simulink model "RealtimeModel"  (Simulink 7.0)
settings: Solver=FixedStepDiscrete  SolverMode=MultiTasking  StartTime=0.0  StopTime=RunningTime  FixedStep=sample  RelTol=1e-3
values from neighbouring files (symbols this model uses):
  Integrator = InitializeIntegrator(Integrator, Structure)    [RealtimeModel_Setup.m]
  Interpolations = SampleRate/sample    [RealtimeModel_Setup.m]
  sample = 1/1024    (= 0.0009765625)    [RealtimeModel_Setup.m]
  SampleRate = Integrator.Timestep    [RealtimeModel_Setup.m]
undefined symbols (not defined in the file or in its folder): Elements
(part 1 of 3)
CloseFcn:
  | rtwprivate ssgencode ModelCloseRequest hybriddaq1dof
settings Model: MinMaxOverflowLogging=ForceOff  Creator=NEESsim1  LastModifiedBy=Tommy  BufferReuse=off
settings OptimizationCC: BlockReduction=off  OptimizeBlockIOStorage=off  BufferReuse=off  ExpressionFolding=off  LocalBlockOutputs=off
settings DebuggingCC: SignalResolutionControl=TryResolveAllWithWarning  MultiTaskDSMMsg=warning  StrictBusMsg=ErrorLevel1
settings RTWCC: SystemTargetFile=xpctarget.tlc  TemplateMakefile=xpc_default_tmf  Description=xPC Target  ProcessScript=xpctarget_make_rtw_hook
settings xpcTargetCC: TargetFcnLib=ansi_tfl_tmw.mat  GenFloatMathFcnCalls=ANSI_C  CompOptLevelCompliant=off  PortableWordSizes=off
settings CustomProperty: DataType=string  Value=Real-Time

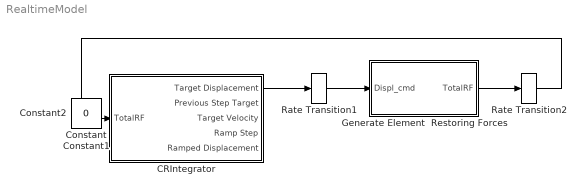
== system RealtimeModel ==
  CRIntegrator : Subsystem
  Generate Element  Restoring Forces : Subsystem  TreatAsAtomicUnit=on  SystemSampleTime=SampleRate
  Rate Transition1 : RateTransition  Deterministic=off
  Rate Transition2 : RateTransition  Deterministic=off
  Constant : Constant  IOType=siggen  Value=0  OutDataType=sfix(16)  OutScaling=2^0
  Constant1 : Constant  IOType=siggen  Value=0  OutDataType=sfix(16)  OutScaling=2^0
  Constant2 : Constant  IOType=siggen  Value=0  OutDataType=sfix(16)  OutScaling=2^0
  wires:
  Rate Transition1/1 -> Generate Element  Restoring Forces/1(Displ_cmd)
  Generate Element  Restoring Forces/1(TotalRF) -> Rate Transition2/1
  CRIntegrator/1(Target Displacement) -> Rate Transition1/1
  Rate Transition2/1 -> CRIntegrator/1(TotalRF)

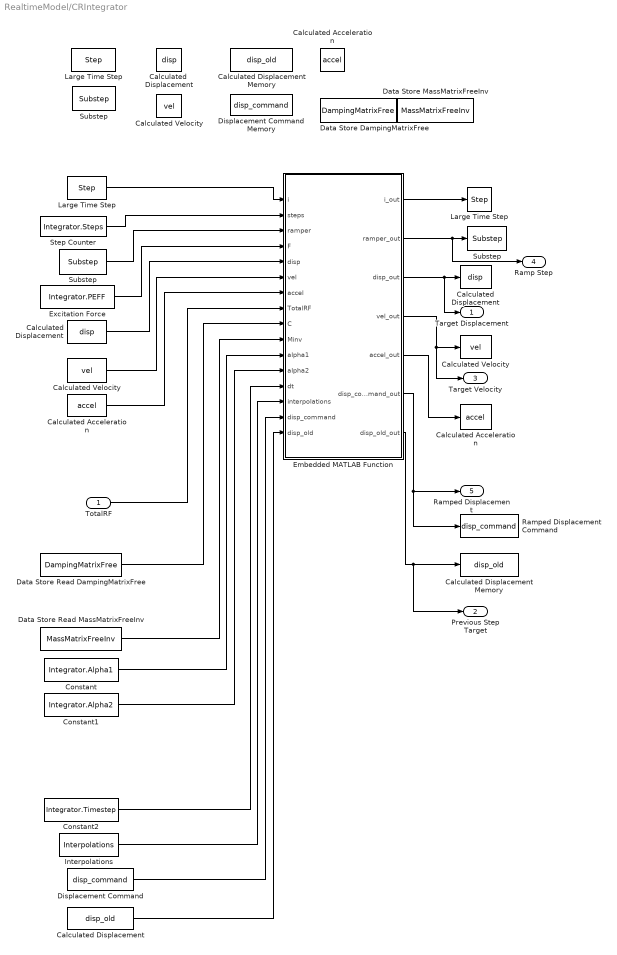
== system RealtimeModel/CRIntegrator ==
  TotalRF : Inport  OutDataType=sfix(16)  OutScaling=2^0
  " Calculated Acceleration" : DataStoreWrite  DataStoreName=accel  SampleTime=sample
  " Calculated Displacement" : DataStoreWrite  DataStoreName=disp  SampleTime=sample
  " Calculated Displacement Memory" : DataStoreWrite  DataStoreName=disp_old  SampleTime=sample
  " Calculated Velocity" : DataStoreWrite  DataStoreName=vel  SampleTime=sample
  " Large Time Step" : DataStoreWrite  DataStoreName=Step  SampleTime=sample
  " Substep" : DataStoreWrite  DataStoreName=Substep  SampleTime=sample
  Calculated Acceleration : DataStoreMemory  DataStoreName=accel  InitialValue=Integrator.Acceleration  OutDataType=sfix(16)  OutScaling=2^0
  Calculated Velocity : DataStoreMemory  DataStoreName=vel  InitialValue=Integrator.Velocity  OutDataType=sfix(16)  OutScaling=2^0
  Calculated  Displacement : DataStoreMemory  DataStoreName=disp  InitialValue=Integrator.Displacement  OutDataType=sfix(16)  OutScaling=2^0
  "Calculated Acceleration " : DataStoreRead  DataStoreName=accel  SampleTime=sample
  Calculated Displacement : DataStoreRead  DataStoreName=disp_old  SampleTime=sample
  Calculated Displacement Memory : DataStoreMemory  DataStoreName=disp_old  InitialValue=Integrator.Displacement  OutDataType=sfix(16)  OutScaling=2^0
  "Calculated Displacement " : DataStoreRead  DataStoreName=disp  SampleTime=sample
  "Calculated Velocity " : DataStoreRead  DataStoreName=vel  SampleTime=sample
  Constant : Constant  Value=Integrator.Alpha1  OutDataType=sfix(16)  OutScaling=2^0
  Constant1 : Constant  Value=Integrator.Alpha2  OutDataType=sfix(16)  OutScaling=2^0
  Constant2 : Constant  Value=Integrator.Timestep  OutDataType=sfix(16)  OutScaling=2^0
  Data Store DampingMatrixFree : DataStoreMemory  DataStoreName=DampingMatrixFree  InitialValue=Structure.DampingMatrixFree  OutDataType=sfix(16)  OutScaling=2^0
  Data Store MassMatrixFreeInv : DataStoreMemory  DataStoreName=MassMatrixFreeInv  InitialValue=Structure.MassMatrixFreeInv  OutDataType=sfix(16)  OutScaling=2^0
  Data Store Read DampingMatrixFree : DataStoreRead  DataStoreName=DampingMatrixFree  SampleTime=sample
  Data Store Read MassMatrixFreeInv : DataStoreRead  DataStoreName=MassMatrixFreeInv  SampleTime=sample
  Displacement Command Memory : DataStoreMemory  DataStoreName=disp_command  InitialValue=Integrator.Displacement  OutDataType=sfix(16)  OutScaling=2^0
  "Displacement Command " : DataStoreRead  DataStoreName=disp_command  SampleTime=sample
  Embedded MATLAB Function : Stateflow chart
  Excitation Force : Constant  Value=Integrator.PEFF  OutDataType=sfix(16)  OutScaling=2^0
  Interpolations : Constant  Value=Interpolations  OutDataType=sfix(16)  OutScaling=2^0  SampleTime=sample
  Large Time Step : DataStoreMemory  DataStoreName=Step  OutDataType=sfix(16)  OutScaling=2^0
  "Large Time Step " : DataStoreRead  DataStoreName=Step  SampleTime=sample
  Ramped Displacement Command : DataStoreWrite  DataStoreName=disp_command  SampleTime=sample
  Step Counter : Constant  Value=Integrator.Steps  OutDataType=sfix(16)  OutScaling=2^0  SampleTime=sample
  Substep : DataStoreMemory  DataStoreName=Substep  InitialValue=1  OutDataType=sfix(16)  OutScaling=2^0
  "Substep " : DataStoreRead  DataStoreName=Substep  SampleTime=sample
  Target Displacement : Outport  OutDataType=sfix(16)  OutScaling=2^0
  Previous Step Target : Outport  Port=2  OutDataType=sfix(16)  OutScaling=2^0
  Target Velocity : Outport  Port=3  OutDataType=sfix(16)  OutScaling=2^0
  Ramp Step : Outport  Port=4  OutDataType=sfix(16)  OutScaling=2^0
  Ramped Displacement : Outport  Port=5  OutDataType=sfix(16)  OutScaling=2^0
  wires:
  Excitation Force/1 -> Embedded MATLAB Function/4(F)
  Calculated Displacement/1 -> Embedded MATLAB Function/16(disp_old)
  "Displacement Command "/1 -> Embedded MATLAB Function/15(disp_command)
  "Calculated Acceleration "/1 -> Embedded MATLAB Function/7(accel)
  "Calculated Velocity "/1 -> Embedded MATLAB Function/6(vel)
  "Calculated Displacement "/1 -> Embedded MATLAB Function/5(disp)
  "Substep "/1 -> Embedded MATLAB Function/3(ramper)
  Embedded MATLAB Function/7(disp_old_out) -> Previous Step Target/1, " Calculated Displacement Memory"/1
  Embedded MATLAB Function/5(accel_out) -> " Calculated Acceleration"/1
  Embedded MATLAB Function/3(disp_out) -> " Calculated Displacement"/1, Target Displacement/1
  Embedded MATLAB Function/2(ramper_out) -> Ramp Step/1, " Substep"/1
  Embedded MATLAB Function/1(i_out) -> " Large Time Step"/1
  Constant1/1 -> Embedded MATLAB Function/12(alpha2)
  Constant/1 -> Embedded MATLAB Function/11(alpha1)
  Step Counter/1 -> Embedded MATLAB Function/2(steps)
  Constant2/1 -> Embedded MATLAB Function/13(dt)
  TotalRF/1 -> Embedded MATLAB Function/8(TotalRF)
  Embedded MATLAB Function/6(disp_command_out) -> Ramped Displacement Command/1, Ramped Displacement/1
  Embedded MATLAB Function/4(vel_out) -> " Calculated Velocity"/1, Target Velocity/1
  Interpolations/1 -> Embedded MATLAB Function/14(interpolations)
  Data Store Read MassMatrixFreeInv/1 -> Embedded MATLAB Function/10(Minv)
  Data Store Read DampingMatrixFree/1 -> Embedded MATLAB Function/9(C)
  "Large Time Step "/1 -> Embedded MATLAB Function/1(i)

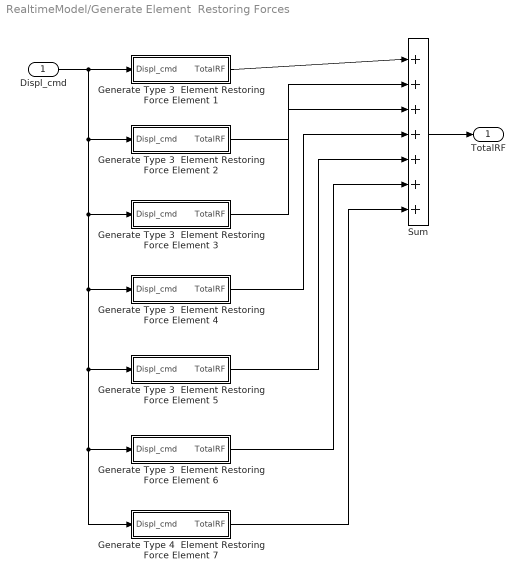
== system RealtimeModel/Generate Element  Restoring Forces ==
  Displ_cmd : Inport  OutDataType=sfix(16)  OutScaling=2^0
  Generate Type 3  Element Restoring Force Element 1 : Subsystem  TreatAsAtomicUnit=on  SystemSampleTime=SampleRate  mask(Generate Type 3 Element Restoring Force){id=1}
      mask prompts: id "Element ID"
      mask help:
      | Generates the Restoring Force vector for a Type 3 Element
      |
      | Enter the ID for this element corresponding with the input configuration file
  Generate Type 3  Element Restoring Force Element 2 : Subsystem  TreatAsAtomicUnit=on  SystemSampleTime=SampleRate  mask(Generate Type 3 Element Restoring Force){id=2}
      mask prompts: id "Element ID"
      mask help:
      | Generates the Restoring Force vector for a Type 3 Element
      |
      | Enter the ID for this element corresponding with the input configuration file
  Generate Type 3  Element Restoring Force Element 3 : Subsystem  TreatAsAtomicUnit=on  SystemSampleTime=SampleRate  mask(Generate Type 3 Element Restoring Force){id=3}
      mask prompts: id "Element ID"
      mask help:
      | Generates the Restoring Force vector for a Type 3 Element
      |
      | Enter the ID for this element corresponding with the input configuration file
  Generate Type 3  Element Restoring Force Element 4 : Subsystem  TreatAsAtomicUnit=on  SystemSampleTime=SampleRate  mask(Generate Type 3 Element Restoring Force){id=4}
      mask prompts: id "Element ID"
      mask help:
      | Generates the Restoring Force vector for a Type 3 Element
      |
      | Enter the ID for this element corresponding with the input configuration file
  Generate Type 3  Element Restoring Force Element 5 : Subsystem  TreatAsAtomicUnit=on  SystemSampleTime=SampleRate  mask(Generate Type 3 Element Restoring Force){id=5}
      mask prompts: id "Element ID"
      mask help:
      | Generates the Restoring Force vector for a Type 3 Element
      |
      | Enter the ID for this element corresponding with the input configuration file
  Generate Type 3  Element Restoring Force Element 6 : Subsystem  TreatAsAtomicUnit=on  SystemSampleTime=SampleRate  mask(Generate Type 3 Element Restoring Force){id=6}
      mask prompts: id "Element ID"
      mask help:
      | Generates the Restoring Force vector for a Type 3 Element
      |
      | Enter the ID for this element corresponding with the input configuration file
  Generate Type 4  Element Restoring Force Element 7 : Subsystem  TreatAsAtomicUnit=on  SystemSampleTime=SampleRate  mask(Generate Type 4 Element Restoring Force){id=7}
      mask prompts: id "Element ID"
      mask help:
      | Generates the Restoring Force vector for a Type 4 Element
      |
      | Enter the ID for this element corresponding with the input configuration file
  Sum : Sum  Inputs=|+++++++  OutDataType=sfix(16)  OutScaling=2^0
  TotalRF : Outport  OutDataType=sfix(16)  OutScaling=2^0
  wires:
  Displ_cmd/1 -> Generate Type 3  Element Restoring Force Element 1/1(Displ_cmd), Generate Type 3  Element Restoring Force Element 2/1(Displ_cmd), Generate Type 3  Element Restoring Force Element 3/1(Displ_cmd), Generate Type 3  Element Restoring Force Element 4/1(Displ_cmd), Generate Type 3  Element Restoring Force Element 5/1(Displ_cmd), Generate Type 3  Element Restoring Force Element 6/1(Displ_cmd), Generate Type 4  Element Restoring Force Element 7/1(Displ_cmd)
  Sum/1 -> TotalRF/1
  Generate Type 3  Element Restoring Force Element 1/1(TotalRF) -> Sum/1
  Generate Type 3  Element Restoring Force Element 2/1(TotalRF) -> Sum/2
  Generate Type 3  Element Restoring Force Element 3/1(TotalRF) -> Sum/3
  Generate Type 3  Element Restoring Force Element 4/1(TotalRF) -> Sum/4
  Generate Type 3  Element Restoring Force Element 5/1(TotalRF) -> Sum/5
  Generate Type 3  Element Restoring Force Element 6/1(TotalRF) -> Sum/6
  Generate Type 4  Element Restoring Force Element 7/1(TotalRF) -> Sum/7

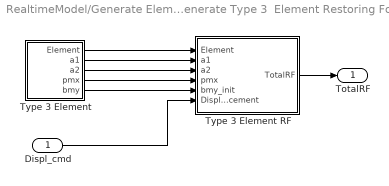
== system RealtimeModel/Generate Element  Restoring Forces/Generate Type 3  Element Restoring Force Element 1 ==
  Displ_cmd : Inport  OutDataType=sfix(16)  OutScaling=2^0
  "Type 3 Element " : Subsystem  mask(Element Type 3){id=id}
      mask prompts: id "Element ID:"
      mask help: Enter the ID for this element corresponding with the input configuration file
  Type 3 Element RF : Stateflow chart  TreatAsAtomicUnit=on  SystemSampleTime=SampleRate
  TotalRF : Outport  OutDataType=sfix(16)  OutScaling=2^0
  wires:
  Displ_cmd/1 -> Type 3 Element RF/6(Displacement)
  "Type 3 Element "/1(Element) -> Type 3 Element RF/1(Element)
  Type 3 Element RF/1(TotalRF) -> TotalRF/1
  "Type 3 Element "/2(a1) -> Type 3 Element RF/2(a1)
  "Type 3 Element "/3(a2) -> Type 3 Element RF/3(a2)
  "Type 3 Element "/4(pmx) -> Type 3 Element RF/4(pmx)
  "Type 3 Element "/5(bmy) -> Type 3 Element RF/5(bmy_init)

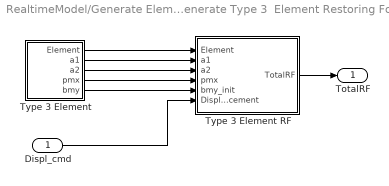
== system RealtimeModel/Generate Element  Restoring Forces/Generate Type 3  Element Restoring Force Element 2 ==
  Displ_cmd : Inport  OutDataType=sfix(16)  OutScaling=2^0
  "Type 3 Element " : Subsystem  mask(Element Type 3){id=id}
      mask prompts: id "Element ID:"
      mask help: Enter the ID for this element corresponding with the input configuration file
  Type 3 Element RF : Stateflow chart  TreatAsAtomicUnit=on  SystemSampleTime=SampleRate
  TotalRF : Outport  OutDataType=sfix(16)  OutScaling=2^0
  wires:
  "Type 3 Element "/5(bmy) -> Type 3 Element RF/5(bmy_init)
  "Type 3 Element "/4(pmx) -> Type 3 Element RF/4(pmx)
  "Type 3 Element "/3(a2) -> Type 3 Element RF/3(a2)
  "Type 3 Element "/2(a1) -> Type 3 Element RF/2(a1)
  Type 3 Element RF/1(TotalRF) -> TotalRF/1
  "Type 3 Element "/1(Element) -> Type 3 Element RF/1(Element)
  Displ_cmd/1 -> Type 3 Element RF/6(Displacement)

== system RealtimeModel/Generate Element  Restoring Forces/Generate Type 3  Element Restoring Force Element 3 ==
  Displ_cmd : Inport  OutDataType=sfix(16)  OutScaling=2^0
  "Type 3 Element " : Subsystem  mask(Element Type 3){id=id}
      mask prompts: id "Element ID:"
      mask help: Enter the ID for this element corresponding with the input configuration file
  Type 3 Element RF : Stateflow chart  TreatAsAtomicUnit=on  SystemSampleTime=SampleRate
  TotalRF : Outport  OutDataType=sfix(16)  OutScaling=2^0
  wires:
  "Type 3 Element "/5(bmy) -> Type 3 Element RF/5(bmy_init)
  "Type 3 Element "/4(pmx) -> Type 3 Element RF/4(pmx)
  "Type 3 Element "/3(a2) -> Type 3 Element RF/3(a2)
  "Type 3 Element "/2(a1) -> Type 3 Element RF/2(a1)
  Type 3 Element RF/1(TotalRF) -> TotalRF/1
  "Type 3 Element "/1(Element) -> Type 3 Element RF/1(Element)
  Displ_cmd/1 -> Type 3 Element RF/6(Displacement)

== system RealtimeModel/Generate Element  Restoring Forces/Generate Type 3  Element Restoring Force Element 4 ==
  Displ_cmd : Inport  OutDataType=sfix(16)  OutScaling=2^0
  "Type 3 Element " : Subsystem  mask(Element Type 3){id=id}
      mask prompts: id "Element ID:"
      mask help: Enter the ID for this element corresponding with the input configuration file
  Type 3 Element RF : Stateflow chart  TreatAsAtomicUnit=on  SystemSampleTime=SampleRate
  TotalRF : Outport  OutDataType=sfix(16)  OutScaling=2^0
  wires:
  Displ_cmd/1 -> Type 3 Element RF/6(Displacement)
  "Type 3 Element "/1(Element) -> Type 3 Element RF/1(Element)
  Type 3 Element RF/1(TotalRF) -> TotalRF/1
  "Type 3 Element "/2(a1) -> Type 3 Element RF/2(a1)
  "Type 3 Element "/3(a2) -> Type 3 Element RF/3(a2)
  "Type 3 Element "/4(pmx) -> Type 3 Element RF/4(pmx)
  "Type 3 Element "/5(bmy) -> Type 3 Element RF/5(bmy_init)

== system RealtimeModel/Generate Element  Restoring Forces/Generate Type 3  Element Restoring Force Element 5 ==
  Displ_cmd : Inport  OutDataType=sfix(16)  OutScaling=2^0
  "Type 3 Element " : Subsystem  mask(Element Type 3){id=id}
      mask prompts: id "Element ID:"
      mask help: Enter the ID for this element corresponding with the input configuration file
  Type 3 Element RF : Stateflow chart  TreatAsAtomicUnit=on  SystemSampleTime=SampleRate
  TotalRF : Outport  OutDataType=sfix(16)  OutScaling=2^0
  wires:
  "Type 3 Element "/5(bmy) -> Type 3 Element RF/5(bmy_init)
  "Type 3 Element "/4(pmx) -> Type 3 Element RF/4(pmx)
  "Type 3 Element "/3(a2) -> Type 3 Element RF/3(a2)
  "Type 3 Element "/2(a1) -> Type 3 Element RF/2(a1)
  Type 3 Element RF/1(TotalRF) -> TotalRF/1
  "Type 3 Element "/1(Element) -> Type 3 Element RF/1(Element)
  Displ_cmd/1 -> Type 3 Element RF/6(Displacement)

== system RealtimeModel/Generate Element  Restoring Forces/Generate Type 3  Element Restoring Force Element 6 ==
  Displ_cmd : Inport  OutDataType=sfix(16)  OutScaling=2^0
  "Type 3 Element " : Subsystem  mask(Element Type 3){id=id}
      mask prompts: id "Element ID:"
      mask help: Enter the ID for this element corresponding with the input configuration file
  Type 3 Element RF : Stateflow chart  TreatAsAtomicUnit=on  SystemSampleTime=SampleRate
  TotalRF : Outport  OutDataType=sfix(16)  OutScaling=2^0
  wires:
  Displ_cmd/1 -> Type 3 Element RF/6(Displacement)
  "Type 3 Element "/1(Element) -> Type 3 Element RF/1(Element)
  Type 3 Element RF/1(TotalRF) -> TotalRF/1
  "Type 3 Element "/2(a1) -> Type 3 Element RF/2(a1)
  "Type 3 Element "/3(a2) -> Type 3 Element RF/3(a2)
  "Type 3 Element "/4(pmx) -> Type 3 Element RF/4(pmx)
  "Type 3 Element "/5(bmy) -> Type 3 Element RF/5(bmy_init)

== system RealtimeModel/Generate Element  Restoring Forces/Generate Type 4  Element Restoring Force Element 7 ==
  Displ_cmd : Inport  OutDataType=sfix(16)  OutScaling=2^0
  "Type 4 Element " : Subsystem  mask(Element Type 4){id=id}
      mask prompts: id "Element ID:"
      mask help: Enter the ID for this element corresponding with the input configuration file
  Type 4 Element RF : Stateflow chart  TreatAsAtomicUnit=on  SystemSampleTime=SampleRate
  TotalRF : Outport  OutDataType=sfix(16)  OutScaling=2^0
  wires:
  "Type 4 Element "/1(Element) -> Type 4 Element RF/1(Element)
  Type 4 Element RF/1(TotalRF) -> TotalRF/1
  Displ_cmd/1 -> Type 4 Element RF/2(Displacement)

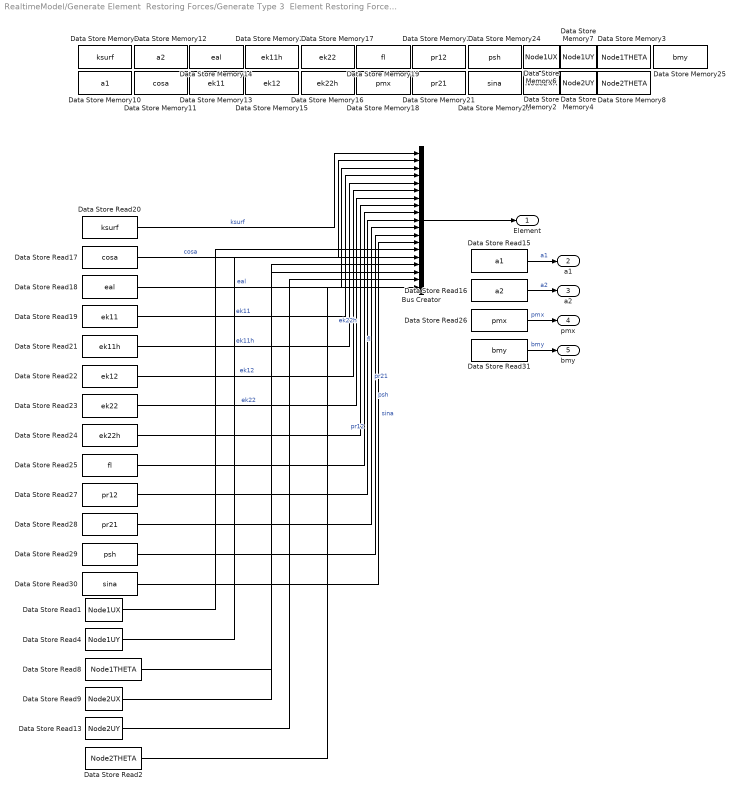
== system RealtimeModel/Generate Element  Restoring Forces/Generate Type 3  Element Restoring Force Element 1/Type 3 Element  ==
  Bus Creator : BusCreator  Inputs=19
  Data Store Memory10 : DataStoreMemory  DataStoreName=a1  InitialValue=Elements{id}.a1  OutDataType=sfix(16)  OutScaling=2^0
  Data Store Memory11 : DataStoreMemory  DataStoreName=cosa  InitialValue=Elements{id}.cosa  OutDataType=sfix(16)  OutScaling=2^0
  Data Store Memory12 : DataStoreMemory  DataStoreName=a2  InitialValue=Elements{id}.a2  OutDataType=sfix(16)  OutScaling=2^0
  Data Store Memory13 : DataStoreMemory  DataStoreName=ek11  InitialValue=Elements{id}.ek11  OutDataType=sfix(16)  OutScaling=2^0
  Data Store Memory14 : DataStoreMemory  DataStoreName=eal  InitialValue=Elements{id}.eal  OutDataType=sfix(16)  OutScaling=2^0
  Data Store Memory15 : DataStoreMemory  DataStoreName=ek12  InitialValue=Elements{id}.ek12  OutDataType=sfix(16)  OutScaling=2^0
  Data Store Memory16 : DataStoreMemory  DataStoreName=ek22h  InitialValue=Elements{id}.ek22h  OutDataType=sfix(16)  OutScaling=2^0
  Data Store Memory17 : DataStoreMemory  DataStoreName=ek22  InitialValue=Elements{id}.ek22  OutDataType=sfix(16)  OutScaling=2^0
  Data Store Memory18 : DataStoreMemory  DataStoreName=pmx  InitialValue=Elements{id}.pmx  OutDataType=sfix(16)  OutScaling=2^0
  Data Store Memory19 : DataStoreMemory  DataStoreName=fl  InitialValue=Elements{id}.fl  OutDataType=sfix(16)  OutScaling=2^0
  Data Store Memory2 : DataStoreMemory  DataStoreName=Node2UX  InitialValue=Elements{id}.Nodes(2).UX  OutDataType=sfix(16)  OutScaling=2^0
  Data Store Memory20 : DataStoreMemory  DataStoreName=ek11h  InitialValue=Elements{id}.ek11h  OutDataType=sfix(16)  OutScaling=2^0
  Data Store Memory21 : DataStoreMemory  DataStoreName=pr21  InitialValue=Elements{id}.pr21  OutDataType=sfix(16)  OutScaling=2^0
  Data Store Memory22 : DataStoreMemory  DataStoreName=pr12  InitialValue=Elements{id}.pr12  OutDataType=sfix(16)  OutScaling=2^0
  Data Store Memory23 : DataStoreMemory  DataStoreName=sina  InitialValue=Elements{id}.sina  OutDataType=sfix(16)  OutScaling=2^0
  Data Store Memory24 : DataStoreMemory  DataStoreName=psh  InitialValue=Elements{id}.psh  OutDataType=sfix(16)  OutScaling=2^0
  Data Store Memory25 : DataStoreMemory  DataStoreName=bmy  InitialValue=Elements{id}.bmy  OutDataType=sfix(16)  OutScaling=2^0
  Data Store Memory3 : DataStoreMemory  DataStoreName=Node1THETA  InitialValue=Elements{id}.Nodes(1).THETA  OutDataType=sfix(16)  OutScaling=2^0
  Data Store Memory4 : DataStoreMemory  DataStoreName=Node2UY  InitialValue=Elements{id}.Nodes(2).UY  OutDataType=sfix(16)  OutScaling=2^0
  Data Store Memory6 : DataStoreMemory  DataStoreName=Node1UX  InitialValue=Elements{id}.Nodes(1).UX  OutDataType=sfix(16)  OutScaling=2^0
  Data Store Memory7 : DataStoreMemory  DataStoreName=Node1UY  InitialValue=Elements{id}.Nodes(1).UY  OutDataType=sfix(16)  OutScaling=2^0
  Data Store Memory8 : DataStoreMemory  DataStoreName=Node2THETA  InitialValue=Elements{id}.Nodes(2).THETA  OutDataType=sfix(16)  OutScaling=2^0
  Data Store Memory9 : DataStoreMemory  DataStoreName=ksurf  InitialValue=Elements{id}.ksurf  OutDataType=sfix(16)  OutScaling=2^0
  Data Store Read1 : DataStoreRead  DataStoreName=Node1UX  SampleTime=-1
  Data Store Read13 : DataStoreRead  DataStoreName=Node2UY  SampleTime=-1
  Data Store Read15 : DataStoreRead  DataStoreName=a1  SampleTime=-1
  Data Store Read16 : DataStoreRead  DataStoreName=a2  SampleTime=-1
  Data Store Read17 : DataStoreRead  DataStoreName=cosa  SampleTime=-1
  Data Store Read18 : DataStoreRead  DataStoreName=eal  SampleTime=-1
  Data Store Read19 : DataStoreRead  DataStoreName=ek11  SampleTime=-1
  Data Store Read2 : DataStoreRead  DataStoreName=Node2THETA  SampleTime=-1
  Data Store Read20 : DataStoreRead  DataStoreName=ksurf  SampleTime=-1
  Data Store Read21 : DataStoreRead  DataStoreName=ek11h  SampleTime=-1
  Data Store Read22 : DataStoreRead  DataStoreName=ek12  SampleTime=-1
  Data Store Read23 : DataStoreRead  DataStoreName=ek22  SampleTime=-1
  Data Store Read24 : DataStoreRead  DataStoreName=ek22h  SampleTime=-1
  Data Store Read25 : DataStoreRead  DataStoreName=fl  SampleTime=-1
  Data Store Read26 : DataStoreRead  DataStoreName=pmx  SampleTime=-1
  Data Store Read27 : DataStoreRead  DataStoreName=pr12  SampleTime=-1
  Data Store Read28 : DataStoreRead  DataStoreName=pr21  SampleTime=-1
  Data Store Read29 : DataStoreRead  DataStoreName=psh  SampleTime=-1
  Data Store Read30 : DataStoreRead  DataStoreName=sina  SampleTime=-1
  Data Store Read31 : DataStoreRead  DataStoreName=bmy  SampleTime=-1
  Data Store Read4 : DataStoreRead  DataStoreName=Node1UY  SampleTime=-1
  Data Store Read8 : DataStoreRead  DataStoreName=Node1THETA  SampleTime=-1
  Data Store Read9 : DataStoreRead  DataStoreName=Node2UX  SampleTime=-1
  Element : Outport  OutDataType=sfix(16)  OutScaling=2^0
  a1 : Outport  Port=2  OutDataType=sfix(16)  OutScaling=2^0
  a2 : Outport  Port=3  OutDataType=sfix(16)  OutScaling=2^0
  pmx : Outport  Port=4  OutDataType=sfix(16)  OutScaling=2^0
  bmy : Outport  Port=5  OutDataType=sfix(16)  OutScaling=2^0
  wires:
  Data Store Read31/1 -> bmy/1  "bmy"
  Data Store Read26/1 -> pmx/1  "pmx"
  Data Store Read16/1 -> a2/1  "a2"
  Data Store Read15/1 -> a1/1  "a1"
  Data Store Read30/1 -> Bus Creator/13  "sina"
  Data Store Read29/1 -> Bus Creator/12  "psh"
  Data Store Read28/1 -> Bus Creator/11  "pr21"
  Data Store Read27/1 -> Bus Creator/10  "pr12"
  Data Store Read25/1 -> Bus Creator/9  "fl"
  Data Store Read24/1 -> Bus Creator/8  "ek22h"
  Data Store Read23/1 -> Bus Creator/7  "ek22"
  Data Store Read22/1 -> Bus Creator/6  "ek12"
  Data Store Read21/1 -> Bus Creator/5  "ek11h"
  Data Store Read19/1 -> Bus Creator/4  "ek11"
  Data Store Read18/1 -> Bus Creator/3  "eal"
  Data Store Read17/1 -> Bus Creator/2  "cosa"
  Data Store Read20/1 -> Bus Creator/1  "ksurf"
  Bus Creator/1 -> Element/1
  Data Store Read1/1 -> Bus Creator/14
  Data Store Read4/1 -> Bus Creator/15
  Data Store Read8/1 -> Bus Creator/16
  Data Store Read9/1 -> Bus Creator/17
  Data Store Read13/1 -> Bus Creator/18
  Data Store Read2/1 -> Bus Creator/19

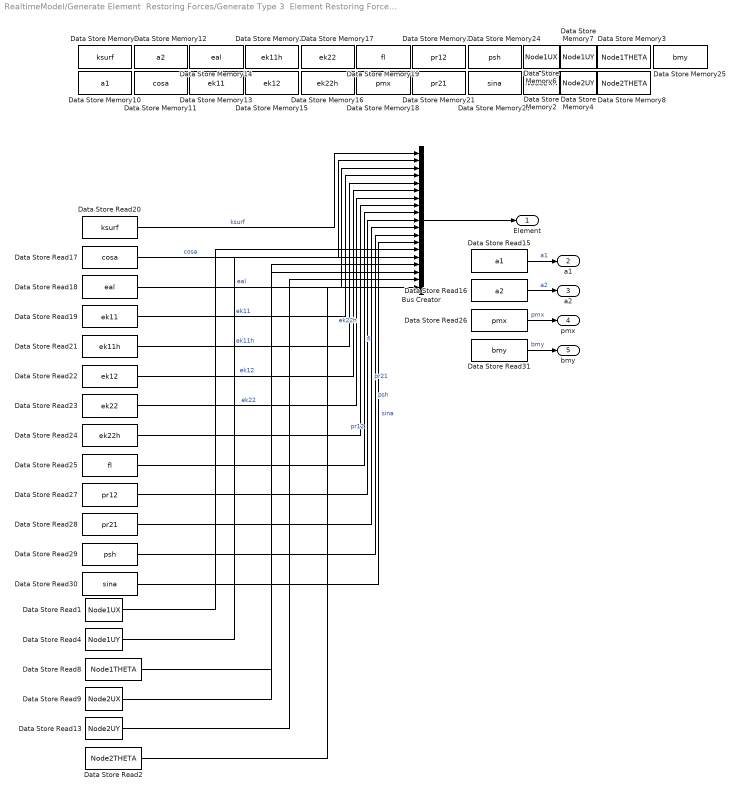
== system RealtimeModel/Generate Element  Restoring Forces/Generate Type 3  Element Restoring Force Element 2/Type 3 Element  ==
  Bus Creator : BusCreator  Inputs=19
  Data Store Memory10 : DataStoreMemory  DataStoreName=a1  InitialValue=Elements{id}.a1  OutDataType=sfix(16)  OutScaling=2^0
  Data Store Memory11 : DataStoreMemory  DataStoreName=cosa  InitialValue=Elements{id}.cosa  OutDataType=sfix(16)  OutScaling=2^0
  Data Store Memory12 : DataStoreMemory  DataStoreName=a2  InitialValue=Elements{id}.a2  OutDataType=sfix(16)  OutScaling=2^0
  Data Store Memory13 : DataStoreMemory  DataStoreName=ek11  InitialValue=Elements{id}.ek11  OutDataType=sfix(16)  OutScaling=2^0
  Data Store Memory14 : DataStoreMemory  DataStoreName=eal  InitialValue=Elements{id}.eal  OutDataType=sfix(16)  OutScaling=2^0
  Data Store Memory15 : DataStoreMemory  DataStoreName=ek12  InitialValue=Elements{id}.ek12  OutDataType=sfix(16)  OutScaling=2^0
  Data Store Memory16 : DataStoreMemory  DataStoreName=ek22h  InitialValue=Elements{id}.ek22h  OutDataType=sfix(16)  OutScaling=2^0
  Data Store Memory17 : DataStoreMemory  DataStoreName=ek22  InitialValue=Elements{id}.ek22  OutDataType=sfix(16)  OutScaling=2^0
  Data Store Memory18 : DataStoreMemory  DataStoreName=pmx  InitialValue=Elements{id}.pmx  OutDataType=sfix(16)  OutScaling=2^0
  Data Store Memory19 : DataStoreMemory  DataStoreName=fl  InitialValue=Elements{id}.fl  OutDataType=sfix(16)  OutScaling=2^0
  Data Store Memory2 : DataStoreMemory  DataStoreName=Node2UX  InitialValue=Elements{id}.Nodes(2).UX  OutDataType=sfix(16)  OutScaling=2^0
  Data Store Memory20 : DataStoreMemory  DataStoreName=ek11h  InitialValue=Elements{id}.ek11h  OutDataType=sfix(16)  OutScaling=2^0
  Data Store Memory21 : DataStoreMemory  DataStoreName=pr21  InitialValue=Elements{id}.pr21  OutDataType=sfix(16)  OutScaling=2^0
  Data Store Memory22 : DataStoreMemory  DataStoreName=pr12  InitialValue=Elements{id}.pr12  OutDataType=sfix(16)  OutScaling=2^0
  Data Store Memory23 : DataStoreMemory  DataStoreName=sina  InitialValue=Elements{id}.sina  OutDataType=sfix(16)  OutScaling=2^0
  Data Store Memory24 : DataStoreMemory  DataStoreName=psh  InitialValue=Elements{id}.psh  OutDataType=sfix(16)  OutScaling=2^0
  Data Store Memory25 : DataStoreMemory  DataStoreName=bmy  InitialValue=Elements{id}.bmy  OutDataType=sfix(16)  OutScaling=2^0
  Data Store Memory3 : DataStoreMemory  DataStoreName=Node1THETA  InitialValue=Elements{id}.Nodes(1).THETA  OutDataType=sfix(16)  OutScaling=2^0
  Data Store Memory4 : DataStoreMemory  DataStoreName=Node2UY  InitialValue=Elements{id}.Nodes(2).UY  OutDataType=sfix(16)  OutScaling=2^0
  Data Store Memory6 : DataStoreMemory  DataStoreName=Node1UX  InitialValue=Elements{id}.Nodes(1).UX  OutDataType=sfix(16)  OutScaling=2^0
  Data Store Memory7 : DataStoreMemory  DataStoreName=Node1UY  InitialValue=Elements{id}.Nodes(1).UY  OutDataType=sfix(16)  OutScaling=2^0
  Data Store Memory8 : DataStoreMemory  DataStoreName=Node2THETA  InitialValue=Elements{id}.Nodes(2).THETA  OutDataType=sfix(16)  OutScaling=2^0
  Data Store Memory9 : DataStoreMemory  DataStoreName=ksurf  InitialValue=Elements{id}.ksurf  OutDataType=sfix(16)  OutScaling=2^0
  Data Store Read1 : DataStoreRead  DataStoreName=Node1UX  SampleTime=-1
  Data Store Read13 : DataStoreRead  DataStoreName=Node2UY  SampleTime=-1
  Data Store Read15 : DataStoreRead  DataStoreName=a1  SampleTime=-1
  Data Store Read16 : DataStoreRead  DataStoreName=a2  SampleTime=-1
  Data Store Read17 : DataStoreRead  DataStoreName=cosa  SampleTime=-1
  Data Store Read18 : DataStoreRead  DataStoreName=eal  SampleTime=-1
  Data Store Read19 : DataStoreRead  DataStoreName=ek11  SampleTime=-1
  Data Store Read2 : DataStoreRead  DataStoreName=Node2THETA  SampleTime=-1
  Data Store Read20 : DataStoreRead  DataStoreName=ksurf  SampleTime=-1
  Data Store Read21 : DataStoreRead  DataStoreName=ek11h  SampleTime=-1
  Data Store Read22 : DataStoreRead  DataStoreName=ek12  SampleTime=-1
  Data Store Read23 : DataStoreRead  DataStoreName=ek22  SampleTime=-1
  Data Store Read24 : DataStoreRead  DataStoreName=ek22h  SampleTime=-1
  Data Store Read25 : DataStoreRead  DataStoreName=fl  SampleTime=-1
  Data Store Read26 : DataStoreRead  DataStoreName=pmx  SampleTime=-1
  Data Store Read27 : DataStoreRead  DataStoreName=pr12  SampleTime=-1
  Data Store Read28 : DataStoreRead  DataStoreName=pr21  SampleTime=-1
  Data Store Read29 : DataStoreRead  DataStoreName=psh  SampleTime=-1
  Data Store Read30 : DataStoreRead  DataStoreName=sina  SampleTime=-1
  Data Store Read31 : DataStoreRead  DataStoreName=bmy  SampleTime=-1
  Data Store Read4 : DataStoreRead  DataStoreName=Node1UY  SampleTime=-1
  Data Store Read8 : DataStoreRead  DataStoreName=Node1THETA  SampleTime=-1
  Data Store Read9 : DataStoreRead  DataStoreName=Node2UX  SampleTime=-1
  Element : Outport  OutDataType=sfix(16)  OutScaling=2^0
  a1 : Outport  Port=2  OutDataType=sfix(16)  OutScaling=2^0
  a2 : Outport  Port=3  OutDataType=sfix(16)  OutScaling=2^0
  pmx : Outport  Port=4  OutDataType=sfix(16)  OutScaling=2^0
  bmy : Outport  Port=5  OutDataType=sfix(16)  OutScaling=2^0
  wires:
  Data Store Read2/1 -> Bus Creator/19
  Data Store Read13/1 -> Bus Creator/18
  Data Store Read9/1 -> Bus Creator/17
  Data Store Read8/1 -> Bus Creator/16
  Data Store Read4/1 -> Bus Creator/15
  Data Store Read1/1 -> Bus Creator/14
  Bus Creator/1 -> Element/1
  Data Store Read20/1 -> Bus Creator/1  "ksurf"
  Data Store Read17/1 -> Bus Creator/2  "cosa"
  Data Store Read18/1 -> Bus Creator/3  "eal"
  Data Store Read19/1 -> Bus Creator/4  "ek11"
  Data Store Read21/1 -> Bus Creator/5  "ek11h"
  Data Store Read22/1 -> Bus Creator/6  "ek12"
  Data Store Read23/1 -> Bus Creator/7  "ek22"
  Data Store Read24/1 -> Bus Creator/8  "ek22h"
  Data Store Read25/1 -> Bus Creator/9  "fl"
  Data Store Read27/1 -> Bus Creator/10  "pr12"
  Data Store Read28/1 -> Bus Creator/11  "pr21"
  Data Store Read29/1 -> Bus Creator/12  "psh"
  Data Store Read30/1 -> Bus Creator/13  "sina"
  Data Store Read15/1 -> a1/1  "a1"
  Data Store Read16/1 -> a2/1  "a2"
  Data Store Read26/1 -> pmx/1  "pmx"
  Data Store Read31/1 -> bmy/1  "bmy"

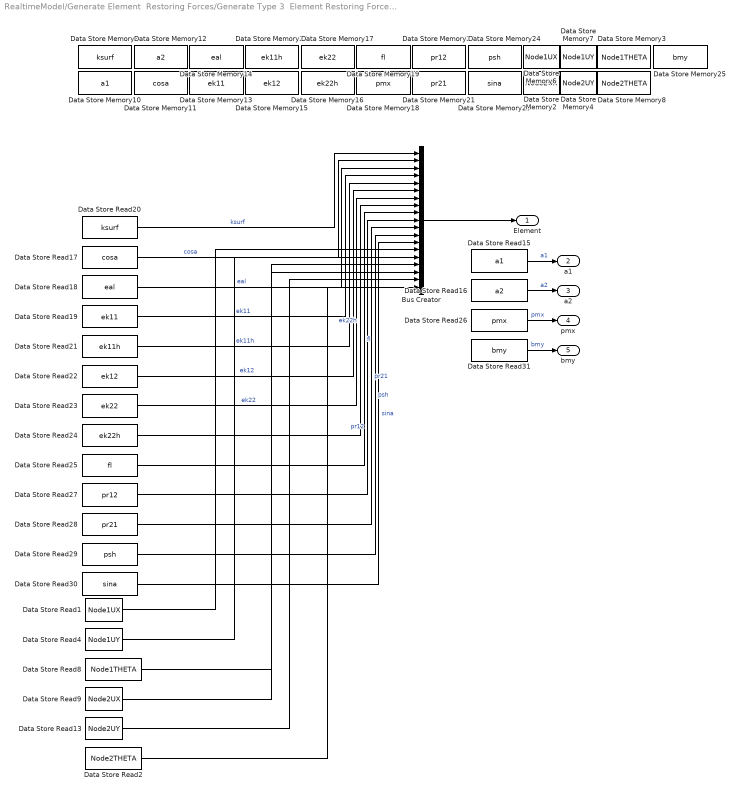
== system RealtimeModel/Generate Element  Restoring Forces/Generate Type 3  Element Restoring Force Element 3/Type 3 Element  ==
  Bus Creator : BusCreator  Inputs=19
  Data Store Memory10 : DataStoreMemory  DataStoreName=a1  InitialValue=Elements{id}.a1  OutDataType=sfix(16)  OutScaling=2^0
  Data Store Memory11 : DataStoreMemory  DataStoreName=cosa  InitialValue=Elements{id}.cosa  OutDataType=sfix(16)  OutScaling=2^0
  Data Store Memory12 : DataStoreMemory  DataStoreName=a2  InitialValue=Elements{id}.a2  OutDataType=sfix(16)  OutScaling=2^0
  Data Store Memory13 : DataStoreMemory  DataStoreName=ek11  InitialValue=Elements{id}.ek11  OutDataType=sfix(16)  OutScaling=2^0
  Data Store Memory14 : DataStoreMemory  DataStoreName=eal  InitialValue=Elements{id}.eal  OutDataType=sfix(16)  OutScaling=2^0
  Data Store Memory15 : DataStoreMemory  DataStoreName=ek12  InitialValue=Elements{id}.ek12  OutDataType=sfix(16)  OutScaling=2^0
  Data Store Memory16 : DataStoreMemory  DataStoreName=ek22h  InitialValue=Elements{id}.ek22h  OutDataType=sfix(16)  OutScaling=2^0
  Data Store Memory17 : DataStoreMemory  DataStoreName=ek22  InitialValue=Elements{id}.ek22  OutDataType=sfix(16)  OutScaling=2^0
  Data Store Memory18 : DataStoreMemory  DataStoreName=pmx  InitialValue=Elements{id}.pmx  OutDataType=sfix(16)  OutScaling=2^0
  Data Store Memory19 : DataStoreMemory  DataStoreName=fl  InitialValue=Elements{id}.fl  OutDataType=sfix(16)  OutScaling=2^0
  Data Store Memory2 : DataStoreMemory  DataStoreName=Node2UX  InitialValue=Elements{id}.Nodes(2).UX  OutDataType=sfix(16)  OutScaling=2^0
  Data Store Memory20 : DataStoreMemory  DataStoreName=ek11h  InitialValue=Elements{id}.ek11h  OutDataType=sfix(16)  OutScaling=2^0
  Data Store Memory21 : DataStoreMemory  DataStoreName=pr21  InitialValue=Elements{id}.pr21  OutDataType=sfix(16)  OutScaling=2^0
  Data Store Memory22 : DataStoreMemory  DataStoreName=pr12  InitialValue=Elements{id}.pr12  OutDataType=sfix(16)  OutScaling=2^0
  Data Store Memory23 : DataStoreMemory  DataStoreName=sina  InitialValue=Elements{id}.sina  OutDataType=sfix(16)  OutScaling=2^0
  Data Store Memory24 : DataStoreMemory  DataStoreName=psh  InitialValue=Elements{id}.psh  OutDataType=sfix(16)  OutScaling=2^0
  Data Store Memory25 : DataStoreMemory  DataStoreName=bmy  InitialValue=Elements{id}.bmy  OutDataType=sfix(16)  OutScaling=2^0
  Data Store Memory3 : DataStoreMemory  DataStoreName=Node1THETA  InitialValue=Elements{id}.Nodes(1).THETA  OutDataType=sfix(16)  OutScaling=2^0
  Data Store Memory4 : DataStoreMemory  DataStoreName=Node2UY  InitialValue=Elements{id}.Nodes(2).UY  OutDataType=sfix(16)  OutScaling=2^0
  Data Store Memory6 : DataStoreMemory  DataStoreName=Node1UX  InitialValue=Elements{id}.Nodes(1).UX  OutDataType=sfix(16)  OutScaling=2^0
  Data Store Memory7 : DataStoreMemory  DataStoreName=Node1UY  InitialValue=Elements{id}.Nodes(1).UY  OutDataType=sfix(16)  OutScaling=2^0
  Data Store Memory8 : DataStoreMemory  DataStoreName=Node2THETA  InitialValue=Elements{id}.Nodes(2).THETA  OutDataType=sfix(16)  OutScaling=2^0
  Data Store Memory9 : DataStoreMemory  DataStoreName=ksurf  InitialValue=Elements{id}.ksurf  OutDataType=sfix(16)  OutScaling=2^0
  Data Store Read1 : DataStoreRead  DataStoreName=Node1UX  SampleTime=-1
  Data Store Read13 : DataStoreRead  DataStoreName=Node2UY  SampleTime=-1
  Data Store Read15 : DataStoreRead  DataStoreName=a1  SampleTime=-1
  Data Store Read16 : DataStoreRead  DataStoreName=a2  SampleTime=-1
  Data Store Read17 : DataStoreRead  DataStoreName=cosa  SampleTime=-1
  Data Store Read18 : DataStoreRead  DataStoreName=eal  SampleTime=-1
  Data Store Read19 : DataStoreRead  DataStoreName=ek11  SampleTime=-1
  Data Store Read2 : DataStoreRead  DataStoreName=Node2THETA  SampleTime=-1
  Data Store Read20 : DataStoreRead  DataStoreName=ksurf  SampleTime=-1
  Data Store Read21 : DataStoreRead  DataStoreName=ek11h  SampleTime=-1
  Data Store Read22 : DataStoreRead  DataStoreName=ek12  SampleTime=-1
  Data Store Read23 : DataStoreRead  DataStoreName=ek22  SampleTime=-1
  Data Store Read24 : DataStoreRead  DataStoreName=ek22h  SampleTime=-1
  Data Store Read25 : DataStoreRead  DataStoreName=fl  SampleTime=-1
  Data Store Read26 : DataStoreRead  DataStoreName=pmx  SampleTime=-1
  Data Store Read27 : DataStoreRead  DataStoreName=pr12  SampleTime=-1
  Data Store Read28 : DataStoreRead  DataStoreName=pr21  SampleTime=-1
  Data Store Read29 : DataStoreRead  DataStoreName=psh  SampleTime=-1
  Data Store Read30 : DataStoreRead  DataStoreName=sina  SampleTime=-1
  Data Store Read31 : DataStoreRead  DataStoreName=bmy  SampleTime=-1
  Data Store Read4 : DataStoreRead  DataStoreName=Node1UY  SampleTime=-1
  Data Store Read8 : DataStoreRead  DataStoreName=Node1THETA  SampleTime=-1
  Data Store Read9 : DataStoreRead  DataStoreName=Node2UX  SampleTime=-1
  Element : Outport  OutDataType=sfix(16)  OutScaling=2^0
  a1 : Outport  Port=2  OutDataType=sfix(16)  OutScaling=2^0
  a2 : Outport  Port=3  OutDataType=sfix(16)  OutScaling=2^0
  pmx : Outport  Port=4  OutDataType=sfix(16)  OutScaling=2^0
  bmy : Outport  Port=5  OutDataType=sfix(16)  OutScaling=2^0
  wires:
  Data Store Read2/1 -> Bus Creator/19
  Data Store Read13/1 -> Bus Creator/18
  Data Store Read9/1 -> Bus Creator/17
  Data Store Read8/1 -> Bus Creator/16
  Data Store Read4/1 -> Bus Creator/15
  Data Store Read1/1 -> Bus Creator/14
  Bus Creator/1 -> Element/1
  Data Store Read20/1 -> Bus Creator/1  "ksurf"
  Data Store Read17/1 -> Bus Creator/2  "cosa"
  Data Store Read18/1 -> Bus Creator/3  "eal"
  Data Store Read19/1 -> Bus Creator/4  "ek11"
  Data Store Read21/1 -> Bus Creator/5  "ek11h"
  Data Store Read22/1 -> Bus Creator/6  "ek12"
  Data Store Read23/1 -> Bus Creator/7  "ek22"
  Data Store Read24/1 -> Bus Creator/8  "ek22h"
  Data Store Read25/1 -> Bus Creator/9  "fl"
  Data Store Read27/1 -> Bus Creator/10  "pr12"
  Data Store Read28/1 -> Bus Creator/11  "pr21"
  Data Store Read29/1 -> Bus Creator/12  "psh"
  Data Store Read30/1 -> Bus Creator/13  "sina"
  Data Store Read15/1 -> a1/1  "a1"
  Data Store Read16/1 -> a2/1  "a2"
  Data Store Read26/1 -> pmx/1  "pmx"
  Data Store Read31/1 -> bmy/1  "bmy"

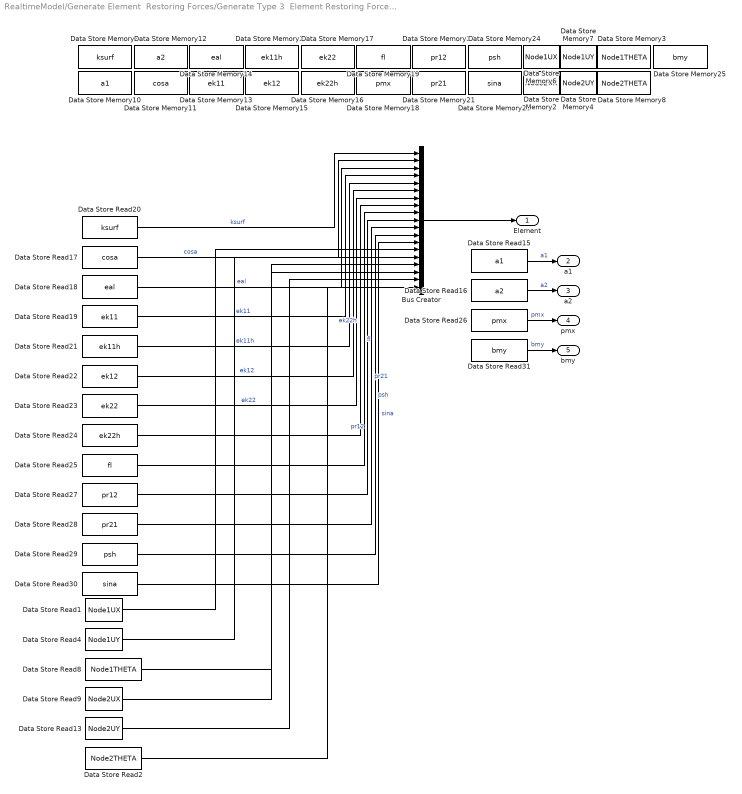
== system RealtimeModel/Generate Element  Restoring Forces/Generate Type 3  Element Restoring Force Element 4/Type 3 Element  ==
  Bus Creator : BusCreator  Inputs=19
  Data Store Memory10 : DataStoreMemory  DataStoreName=a1  InitialValue=Elements{id}.a1  OutDataType=sfix(16)  OutScaling=2^0
  Data Store Memory11 : DataStoreMemory  DataStoreName=cosa  InitialValue=Elements{id}.cosa  OutDataType=sfix(16)  OutScaling=2^0
  Data Store Memory12 : DataStoreMemory  DataStoreName=a2  InitialValue=Elements{id}.a2  OutDataType=sfix(16)  OutScaling=2^0
  Data Store Memory13 : DataStoreMemory  DataStoreName=ek11  InitialValue=Elements{id}.ek11  OutDataType=sfix(16)  OutScaling=2^0
  Data Store Memory14 : DataStoreMemory  DataStoreName=eal  InitialValue=Elements{id}.eal  OutDataType=sfix(16)  OutScaling=2^0
  Data Store Memory15 : DataStoreMemory  DataStoreName=ek12  InitialValue=Elements{id}.ek12  OutDataType=sfix(16)  OutScaling=2^0
  Data Store Memory16 : DataStoreMemory  DataStoreName=ek22h  InitialValue=Elements{id}.ek22h  OutDataType=sfix(16)  OutScaling=2^0
  Data Store Memory17 : DataStoreMemory  DataStoreName=ek22  InitialValue=Elements{id}.ek22  OutDataType=sfix(16)  OutScaling=2^0
  Data Store Memory18 : DataStoreMemory  DataStoreName=pmx  InitialValue=Elements{id}.pmx  OutDataType=sfix(16)  OutScaling=2^0
  Data Store Memory19 : DataStoreMemory  DataStoreName=fl  InitialValue=Elements{id}.fl  OutDataType=sfix(16)  OutScaling=2^0
  Data Store Memory2 : DataStoreMemory  DataStoreName=Node2UX  InitialValue=Elements{id}.Nodes(2).UX  OutDataType=sfix(16)  OutScaling=2^0
  Data Store Memory20 : DataStoreMemory  DataStoreName=ek11h  InitialValue=Elements{id}.ek11h  OutDataType=sfix(16)  OutScaling=2^0
  Data Store Memory21 : DataStoreMemory  DataStoreName=pr21  InitialValue=Elements{id}.pr21  OutDataType=sfix(16)  OutScaling=2^0
  Data Store Memory22 : DataStoreMemory  DataStoreName=pr12  InitialValue=Elements{id}.pr12  OutDataType=sfix(16)  OutScaling=2^0
  Data Store Memory23 : DataStoreMemory  DataStoreName=sina  InitialValue=Elements{id}.sina  OutDataType=sfix(16)  OutScaling=2^0
  Data Store Memory24 : DataStoreMemory  DataStoreName=psh  InitialValue=Elements{id}.psh  OutDataType=sfix(16)  OutScaling=2^0
  Data Store Memory25 : DataStoreMemory  DataStoreName=bmy  InitialValue=Elements{id}.bmy  OutDataType=sfix(16)  OutScaling=2^0
  Data Store Memory3 : DataStoreMemory  DataStoreName=Node1THETA  InitialValue=Elements{id}.Nodes(1).THETA  OutDataType=sfix(16)  OutScaling=2^0
  Data Store Memory4 : DataStoreMemory  DataStoreName=Node2UY  InitialValue=Elements{id}.Nodes(2).UY  OutDataType=sfix(16)  OutScaling=2^0
  Data Store Memory6 : DataStoreMemory  DataStoreName=Node1UX  InitialValue=Elements{id}.Nodes(1).UX  OutDataType=sfix(16)  OutScaling=2^0
  Data Store Memory7 : DataStoreMemory  DataStoreName=Node1UY  InitialValue=Elements{id}.Nodes(1).UY  OutDataType=sfix(16)  OutScaling=2^0
  Data Store Memory8 : DataStoreMemory  DataStoreName=Node2THETA  InitialValue=Elements{id}.Nodes(2).THETA  OutDataType=sfix(16)  OutScaling=2^0
  Data Store Memory9 : DataStoreMemory  DataStoreName=ksurf  InitialValue=Elements{id}.ksurf  OutDataType=sfix(16)  OutScaling=2^0
  Data Store Read1 : DataStoreRead  DataStoreName=Node1UX  SampleTime=-1
  Data Store Read13 : DataStoreRead  DataStoreName=Node2UY  SampleTime=-1
  Data Store Read15 : DataStoreRead  DataStoreName=a1  SampleTime=-1
  Data Store Read16 : DataStoreRead  DataStoreName=a2  SampleTime=-1
  Data Store Read17 : DataStoreRead  DataStoreName=cosa  SampleTime=-1
  Data Store Read18 : DataStoreRead  DataStoreName=eal  SampleTime=-1
  Data Store Read19 : DataStoreRead  DataStoreName=ek11  SampleTime=-1
  Data Store Read2 : DataStoreRead  DataStoreName=Node2THETA  SampleTime=-1
  Data Store Read20 : DataStoreRead  DataStoreName=ksurf  SampleTime=-1
  Data Store Read21 : DataStoreRead  DataStoreName=ek11h  SampleTime=-1
  Data Store Read22 : DataStoreRead  DataStoreName=ek12  SampleTime=-1
  Data Store Read23 : DataStoreRead  DataStoreName=ek22  SampleTime=-1
  Data Store Read24 : DataStoreRead  DataStoreName=ek22h  SampleTime=-1
  Data Store Read25 : DataStoreRead  DataStoreName=fl  SampleTime=-1
  Data Store Read26 : DataStoreRead  DataStoreName=pmx  SampleTime=-1
  Data Store Read27 : DataStoreRead  DataStoreName=pr12  SampleTime=-1
  Data Store Read28 : DataStoreRead  DataStoreName=pr21  SampleTime=-1
  Data Store Read29 : DataStoreRead  DataStoreName=psh  SampleTime=-1
  Data Store Read30 : DataStoreRead  DataStoreName=sina  SampleTime=-1
  Data Store Read31 : DataStoreRead  DataStoreName=bmy  SampleTime=-1
  Data Store Read4 : DataStoreRead  DataStoreName=Node1UY  SampleTime=-1
  Data Store Read8 : DataStoreRead  DataStoreName=Node1THETA  SampleTime=-1
  Data Store Read9 : DataStoreRead  DataStoreName=Node2UX  SampleTime=-1
  Element : Outport  OutDataType=sfix(16)  OutScaling=2^0
  a1 : Outport  Port=2  OutDataType=sfix(16)  OutScaling=2^0
  a2 : Outport  Port=3  OutDataType=sfix(16)  OutScaling=2^0
  pmx : Outport  Port=4  OutDataType=sfix(16)  OutScaling=2^0
  bmy : Outport  Port=5  OutDataType=sfix(16)  OutScaling=2^0
  wires:
  Data Store Read31/1 -> bmy/1  "bmy"
  Data Store Read26/1 -> pmx/1  "pmx"
  Data Store Read16/1 -> a2/1  "a2"
  Data Store Read15/1 -> a1/1  "a1"
  Data Store Read30/1 -> Bus Creator/13  "sina"
  Data Store Read29/1 -> Bus Creator/12  "psh"
  Data Store Read28/1 -> Bus Creator/11  "pr21"
  Data Store Read27/1 -> Bus Creator/10  "pr12"
  Data Store Read25/1 -> Bus Creator/9  "fl"
  Data Store Read24/1 -> Bus Creator/8  "ek22h"
  Data Store Read23/1 -> Bus Creator/7  "ek22"
  Data Store Read22/1 -> Bus Creator/6  "ek12"
  Data Store Read21/1 -> Bus Creator/5  "ek11h"
  Data Store Read19/1 -> Bus Creator/4  "ek11"
  Data Store Read18/1 -> Bus Creator/3  "eal"
  Data Store Read17/1 -> Bus Creator/2  "cosa"
  Data Store Read20/1 -> Bus Creator/1  "ksurf"
  Bus Creator/1 -> Element/1
  Data Store Read1/1 -> Bus Creator/14
  Data Store Read4/1 -> Bus Creator/15
  Data Store Read8/1 -> Bus Creator/16
  Data Store Read9/1 -> Bus Creator/17
  Data Store Read13/1 -> Bus Creator/18
  Data Store Read2/1 -> Bus Creator/19

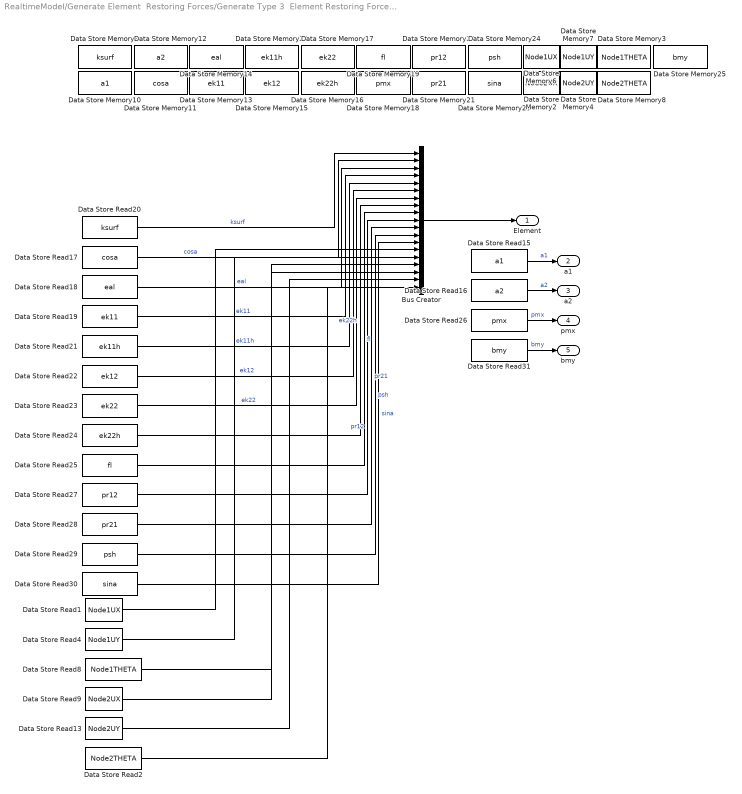
== system RealtimeModel/Generate Element  Restoring Forces/Generate Type 3  Element Restoring Force Element 5/Type 3 Element  ==
  Bus Creator : BusCreator  Inputs=19
  Data Store Memory10 : DataStoreMemory  DataStoreName=a1  InitialValue=Elements{id}.a1  OutDataType=sfix(16)  OutScaling=2^0
  Data Store Memory11 : DataStoreMemory  DataStoreName=cosa  InitialValue=Elements{id}.cosa  OutDataType=sfix(16)  OutScaling=2^0
  Data Store Memory12 : DataStoreMemory  DataStoreName=a2  InitialValue=Elements{id}.a2  OutDataType=sfix(16)  OutScaling=2^0
  Data Store Memory13 : DataStoreMemory  DataStoreName=ek11  InitialValue=Elements{id}.ek11  OutDataType=sfix(16)  OutScaling=2^0
  Data Store Memory14 : DataStoreMemory  DataStoreName=eal  InitialValue=Elements{id}.eal  OutDataType=sfix(16)  OutScaling=2^0
  Data Store Memory15 : DataStoreMemory  DataStoreName=ek12  InitialValue=Elements{id}.ek12  OutDataType=sfix(16)  OutScaling=2^0
  Data Store Memory16 : DataStoreMemory  DataStoreName=ek22h  InitialValue=Elements{id}.ek22h  OutDataType=sfix(16)  OutScaling=2^0
  Data Store Memory17 : DataStoreMemory  DataStoreName=ek22  InitialValue=Elements{id}.ek22  OutDataType=sfix(16)  OutScaling=2^0
  Data Store Memory18 : DataStoreMemory  DataStoreName=pmx  InitialValue=Elements{id}.pmx  OutDataType=sfix(16)  OutScaling=2^0
  Data Store Memory19 : DataStoreMemory  DataStoreName=fl  InitialValue=Elements{id}.fl  OutDataType=sfix(16)  OutScaling=2^0
  Data Store Memory2 : DataStoreMemory  DataStoreName=Node2UX  InitialValue=Elements{id}.Nodes(2).UX  OutDataType=sfix(16)  OutScaling=2^0
  Data Store Memory20 : DataStoreMemory  DataStoreName=ek11h  InitialValue=Elements{id}.ek11h  OutDataType=sfix(16)  OutScaling=2^0
  Data Store Memory21 : DataStoreMemory  DataStoreName=pr21  InitialValue=Elements{id}.pr21  OutDataType=sfix(16)  OutScaling=2^0
  Data Store Memory22 : DataStoreMemory  DataStoreName=pr12  InitialValue=Elements{id}.pr12  OutDataType=sfix(16)  OutScaling=2^0
  Data Store Memory23 : DataStoreMemory  DataStoreName=sina  InitialValue=Elements{id}.sina  OutDataType=sfix(16)  OutScaling=2^0
  Data Store Memory24 : DataStoreMemory  DataStoreName=psh  InitialValue=Elements{id}.psh  OutDataType=sfix(16)  OutScaling=2^0
  Data Store Memory25 : DataStoreMemory  DataStoreName=bmy  InitialValue=Elements{id}.bmy  OutDataType=sfix(16)  OutScaling=2^0
  Data Store Memory3 : DataStoreMemory  DataStoreName=Node1THETA  InitialValue=Elements{id}.Nodes(1).THETA  OutDataType=sfix(16)  OutScaling=2^0
  Data Store Memory4 : DataStoreMemory  DataStoreName=Node2UY  InitialValue=Elements{id}.Nodes(2).UY  OutDataType=sfix(16)  OutScaling=2^0
  Data Store Memory6 : DataStoreMemory  DataStoreName=Node1UX  InitialValue=Elements{id}.Nodes(1).UX  OutDataType=sfix(16)  OutScaling=2^0
  Data Store Memory7 : DataStoreMemory  DataStoreName=Node1UY  InitialValue=Elements{id}.Nodes(1).UY  OutDataType=sfix(16)  OutScaling=2^0
  Data Store Memory8 : DataStoreMemory  DataStoreName=Node2THETA  InitialValue=Elements{id}.Nodes(2).THETA  OutDataType=sfix(16)  OutScaling=2^0
  Data Store Memory9 : DataStoreMemory  DataStoreName=ksurf  InitialValue=Elements{id}.ksurf  OutDataType=sfix(16)  OutScaling=2^0
  Data Store Read1 : DataStoreRead  DataStoreName=Node1UX  SampleTime=-1
  Data Store Read13 : DataStoreRead  DataStoreName=Node2UY  SampleTime=-1
  Data Store Read15 : DataStoreRead  DataStoreName=a1  SampleTime=-1
  Data Store Read16 : DataStoreRead  DataStoreName=a2  SampleTime=-1
  Data Store Read17 : DataStoreRead  DataStoreName=cosa  SampleTime=-1
  Data Store Read18 : DataStoreRead  DataStoreName=eal  SampleTime=-1
  Data Store Read19 : DataStoreRead  DataStoreName=ek11  SampleTime=-1
  Data Store Read2 : DataStoreRead  DataStoreName=Node2THETA  SampleTime=-1
  Data Store Read20 : DataStoreRead  DataStoreName=ksurf  SampleTime=-1
  Data Store Read21 : DataStoreRead  DataStoreName=ek11h  SampleTime=-1
  Data Store Read22 : DataStoreRead  DataStoreName=ek12  SampleTime=-1
  Data Store Read23 : DataStoreRead  DataStoreName=ek22  SampleTime=-1
  Data Store Read24 : DataStoreRead  DataStoreName=ek22h  SampleTime=-1
  Data Store Read25 : DataStoreRead  DataStoreName=fl  SampleTime=-1
  Data Store Read26 : DataStoreRead  DataStoreName=pmx  SampleTime=-1
  Data Store Read27 : DataStoreRead  DataStoreName=pr12  SampleTime=-1
  Data Store Read28 : DataStoreRead  DataStoreName=pr21  SampleTime=-1
  Data Store Read29 : DataStoreRead  DataStoreName=psh  SampleTime=-1
  Data Store Read30 : DataStoreRead  DataStoreName=sina  SampleTime=-1
  Data Store Read31 : DataStoreRead  DataStoreName=bmy  SampleTime=-1
  Data Store Read4 : DataStoreRead  DataStoreName=Node1UY  SampleTime=-1
  Data Store Read8 : DataStoreRead  DataStoreName=Node1THETA  SampleTime=-1
  Data Store Read9 : DataStoreRead  DataStoreName=Node2UX  SampleTime=-1
  Element : Outport  OutDataType=sfix(16)  OutScaling=2^0
  a1 : Outport  Port=2  OutDataType=sfix(16)  OutScaling=2^0
  a2 : Outport  Port=3  OutDataType=sfix(16)  OutScaling=2^0
  pmx : Outport  Port=4  OutDataType=sfix(16)  OutScaling=2^0
  bmy : Outport  Port=5  OutDataType=sfix(16)  OutScaling=2^0
  wires:
  Data Store Read2/1 -> Bus Creator/19
  Data Store Read13/1 -> Bus Creator/18
  Data Store Read9/1 -> Bus Creator/17
  Data Store Read8/1 -> Bus Creator/16
  Data Store Read4/1 -> Bus Creator/15
  Data Store Read1/1 -> Bus Creator/14
  Bus Creator/1 -> Element/1
  Data Store Read20/1 -> Bus Creator/1  "ksurf"
  Data Store Read17/1 -> Bus Creator/2  "cosa"
  Data Store Read18/1 -> Bus Creator/3  "eal"
  Data Store Read19/1 -> Bus Creator/4  "ek11"
  Data Store Read21/1 -> Bus Creator/5  "ek11h"
  Data Store Read22/1 -> Bus Creator/6  "ek12"
  Data Store Read23/1 -> Bus Creator/7  "ek22"
  Data Store Read24/1 -> Bus Creator/8  "ek22h"
  Data Store Read25/1 -> Bus Creator/9  "fl"
  Data Store Read27/1 -> Bus Creator/10  "pr12"
  Data Store Read28/1 -> Bus Creator/11  "pr21"
  Data Store Read29/1 -> Bus Creator/12  "psh"
  Data Store Read30/1 -> Bus Creator/13  "sina"
  Data Store Read15/1 -> a1/1  "a1"
  Data Store Read16/1 -> a2/1  "a2"
  Data Store Read26/1 -> pmx/1  "pmx"
  Data Store Read31/1 -> bmy/1  "bmy"
